simulink model "EBike_Braking"  (R2019b)
settings: Solver=VariableStepAuto  StartTime=0.0  StopTime=1000  MaxStep=0.01  RelTol=1e-3
values from neighbouring files (symbols this model uses):
  A_d = 0.4    [Thesis_Ebike.m]
  Abs = 1    [Thesis_Ebike.m]
  alpha_Conductor = 0.0040    (= 0.004)    [Thesis_Ebike.m]
  Alpha_Magnet = -0.0020    (= -0.002)    [Thesis_Ebike.m]
  Bm = ((Motor_torque_constant)*(17)/(1000*2*pi/60))    (= 0.121753531465)    [Thesis_Ebike.m]
  Braking_Pressure = 100    [Thesis_Ebike.m]
  C_d = 0.9    [Thesis_Ebike.m]
  capacity = 19.5    [Thesis_Ebike.m]
  Coefficient_of_Brake_friction = 0.9    [Thesis_Ebike.m]
  Crank_Length = 0.150    (= 0.15)    [Thesis_Ebike.m]
  Cyclist_weight = 85    [Thesis_Ebike.m]
  Dynamic_Friction_Coefficient = 0.0015    [Thesis_Ebike.m]
  Effective_Radius_of_Disc = 0.16    [Thesis_Ebike.m]
  F_Rider = 100    [Thesis_Ebike.m]
  g = 9.81    [Thesis_Ebike.m]
  Internal_Resistance = 95*10^-3    (= 0.095)    [Thesis_Ebike.m]
  Jm = 10.2 *10^-3    (= 0.0102)    [Thesis_Ebike.m]
  Kb = (51.7/(1000*2*pi/60))    (= 0.493698633471)    [Thesis_Ebike.m]
  L = 0.36*10^-3    (= 0.00036)    [Thesis_Ebike.m]
  Motor_resistance = 88*10^-2    (= 0.88)    [Thesis_Ebike.m]
  Motor_torque_constant = 0.75    [Thesis_Ebike.m]
  Polarization_Capacitance = 1*10^-7    (= 1e-07)    [Thesis_Ebike.m]
  Polarization_Resistance = 95*10^-3    (= 0.095)    [Thesis_Ebike.m]
  Ref_Temp = 25    [Thesis_Ebike.m]
  Rho_air = 1.225    [Thesis_Ebike.m]
  SOC_initial = 100    [Thesis_Ebike.m]
  Static_Friction_Coefficient = 0.0015    [Thesis_Ebike.m]
  Tire_mass = 0.25    [Thesis_Ebike.m]
  Trailer_mass = 50    [Thesis_Ebike.m]
  Vehicle_mass = 25    [Thesis_Ebike.m]
  Wheel_Inertia = 0.0225    [Thesis_Ebike.m]
  Wheel_mass = 0.25    [Thesis_Ebike.m]
  Wheel_Radius = 0.3    [Thesis_Ebike.m]
undefined symbols (not defined in the file or in its folder): sigbuilder_block, V
libraries: simulink x2
(part 3 of 3)

== stateflow chart EBike_Braking/Chart ==
  (junction 5) -> (junction 9) : {signal=1}
  (junction 2) -> (junction 5) [order 1] : [u>850]
  (junction 9) -> (junction 15)
  (default) -> (junction 2)
  (junction 15) -> (junction 18)
  (junction 2) -> (junction 7) [order 2] : [u<850]
  (junction 13) -> (junction 15)
  (junction 7) -> (junction 13) : {signal=0}
  data: u input; signal output

== stateflow chart EBike_Braking/Environmental_Subsystem/Chart ==
  (junction 5) -> (junction 9) : {signal=1}
  (junction 2) -> (junction 5) [order 1] : [u>0]
  (junction 9) -> (junction 15)
  (default) -> (junction 2)
  (junction 15) -> (junction 18)
  (junction 2) -> (junction 7) [order 2] : [u==0]
  (junction 13) -> (junction 15)
  (junction 7) -> (junction 13) : {signal=0}
  data: u input; signal output
